simulink model "Consensus_Demo_03_configuration"  (R2021b)
settings: Solver=VariableStepAuto  StartTime=0.0  StopTime=10.0  RelTol=1e-3
settings Model: Creator=vijay  LastModifiedBy=vijay

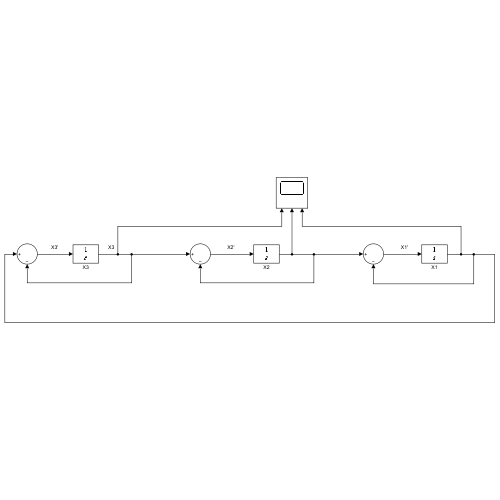
[thumbnail: Simulink's stored preview of the top-level diagram]
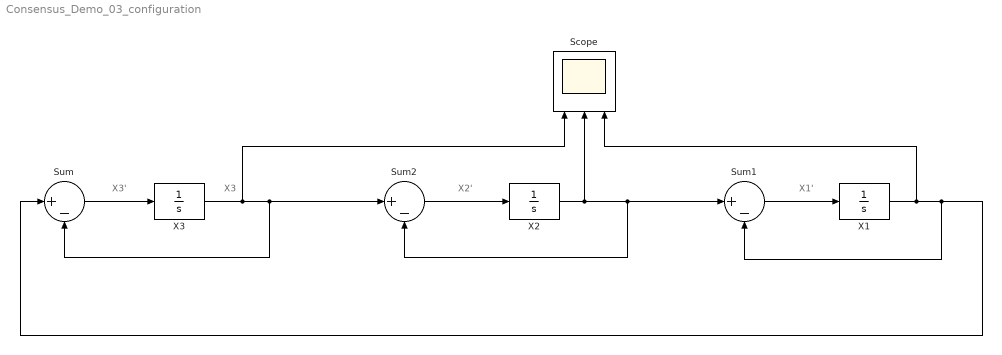
== system Consensus_Demo_03_configuration ==
  note: X3'
  note: X3
  note: X2'
  note: X1'
  Scope : Scope  NumInputPorts=3
  Sum : Sum  Inputs=|+-
  Sum1 : Sum  Inputs=|+-
  Sum2 : Sum  Inputs=|+-
  X1 : Integrator  InitialCondition=0.2
  X2 : Integrator  InitialCondition=0.4
  X3 : Integrator  InitialCondition=0.6
  wires:
  Sum/1 -> X3/1
  X3/1 -> Scope/1, Sum2/1, Sum/2
  Sum2/1 -> X2/1
  X2/1 -> Sum1/1, Sum2/2, Scope/2
  Sum1/1 -> X1/1
  X1/1 -> Scope/3, Sum1/2, Sum/1
